simulink model "car_model_FIXED"  (R2022b)
settings: Solver=VariableStepAuto  StartTime=0.0  StopTime=60  RelTol=1e-3
values from neighbouring files (symbols this model uses):
  ABS_MAX_TORQUE = [25 25 25 25]    [workspace.mat]
  ABS_MAX_TRQ_CMD = 50    [workspace.mat]
  ABS_MIN_TORQUE = [0.01 0.01 0.01 0.01]    [workspace.mat]
  acc_IC = 0    [workspace.mat]
  ACCELERATION_MAX = 30    [workspace.mat]
  ActSuspDutyCycle = 1    [workspace.mat]
  Aeq_left = [0.305756190204 0.308857786592 0.311945941182 0.315020811431 0.318082554689 0.321131328186 0.324167289011 0.327190594103 0.330201400225 0.333199863958 0.336186141681 0.339160389558 ... (261 elements, 1x261)]    [workspace.mat]
  Aeq_right = [-0.961664782545 -0.959835898365 -0.957982924115 -0.956106413788 -0.954206913862 -0.952284963337 -0.950341093764 -0.948375829284 -0.946389686656 -0.944383175301 -0.942356797333 -0.940311047601 ... (261 elements, 1x261)]    [workspace.mat]
  alpha_error = 0.1    [workspace.mat]
  ang_acc_hystersesis = 0.1    [workspace.mat]
  ang_IC = 0    [workspace.mat]
  ang_vel_IC = 0    [workspace.mat]
  area_air = 0.15    [workspace.mat]
  axb = -5    [workspace.mat]
  battery_current_IC = 0    [workspace.mat]
  BATTERY_CURRENT_MAX = 140    [workspace.mat]
  BATTERY_CURRENT_MIN = 0    [workspace.mat]
  battery_FT_IC = 300    [workspace.mat]
  battery_T_IC = 300    [workspace.mat]
  BATTERY_TEMPERATURE_MAX = 60    [workspace.mat]
  BATTERY_TEMPERATURE_MIN = 0    [workspace.mat]
  battery_voltage_IC = 332    [workspace.mat]
  BATTERY_VOLTAGE_MAX = 340    [workspace.mat]
  BATTERY_VOLTAGE_MIN = 60    [workspace.mat]
  br = 0.01    [workspace.mat]
  brake_bias = [0.35 0.35 0.15 0.15]    [workspace.mat]
  Brake_Pressure_IC = 1    [workspace.mat]
  ccl_IC = 0    [workspace.mat]
  CENTER_STEER_ANGLE_MAX = 130    [workspace.mat]
  covarience_matrix_IC = [0.001 0 0 0 0 0 0 0 0 0 0 0 ... (784 elements, 28x28)]    [workspace.mat]
  CURRENT_BUFFER = 25    [workspace.mat]
  cy_sweep = [13568.4166816 14020.2069783 14456.754831 14879.7402576 15289.7264712 15687.2766846 16072.954111 16447.3219632 16810.9434544 17164.3817975 17508.2002054 17842.9618912 ... (101 elements, 1x101)]    [workspace.mat]
  dB = 0.001    [workspace.mat]
  dcl_IC = 140    [workspace.mat]
  DCL_MAX = 130    [workspace.mat]
  DCL_MIN = 0    [workspace.mat]
  deadband_angle = 12    [workspace.mat]
  dIndex = 50    [workspace.mat]
  driver_t = 0.015    [workspace.mat]
  dt_OFF = 4.5    [workspace.mat]
  dt_ON = 7.5    [workspace.mat]
  dTx = 0.01    [workspace.mat]
  dx = 0.1    [workspace.mat]
  dZ = 0.295    [workspace.mat]
  efficiency_grid = [0.759500051293 0.787587791453 0.809832189108 0.826747821898 0.837164543102 0.842744381136 0.842258400104 0.838611650621 0.82826195101 0.814029316176 0.795690627225 0.7759791486 ... (2782 elements, 26x107)]    [workspace.mat]
  F0z = [0 0]    [workspace.mat]
  forward_look_straight = 5    [workspace.mat]
  forward_look_turn = 15    [workspace.mat]
  Fz_IC = 539.55    [workspace.mat]
  Fz_sweep = [200 210 220 230 240 250 260 270 280 290 300 310 ... (101 elements, 1x101)]    [workspace.mat]
  g = 9.81    [workspace.mat]
  GAIN_ABS = 100    [workspace.mat]
  gearbox_efficiency = [0.8 0.8 0.8 0.8]    [workspace.mat]
  gps_counter_IC = 0    [workspace.mat]
  gps_hz = 0.01    [workspace.mat]
  gr = [8.74786324786 8.74786324786 8.74786324786 8.74786324786]    [workspace.mat]
  I = 0    [workspace.mat]
  I_Driver = 1    [workspace.mat]
  indicies = [3 3.5 4 0.5 1 1.5 2 2.5 3 3.5 4 0.5 ... (27 elements, 1x27)]    [workspace.mat]
  IYY = 0.3    [workspace.mat]
  kx_sweep = [8779.958 9178.302 9576.646 9974.99 10373.334 10771.678 11170.022 11568.366 11966.71 12365.054 12763.398 13161.742 ... (101 elements, 1x101)]    [workspace.mat]
  l = [0.772 0.772]    [workspace.mat]
  lambda_star = 0.15    [workspace.mat]
  low_V_SA = 0.001    [workspace.mat]
  lr = 35    [workspace.mat]
  m_all = 220    [workspace.mat]
  m_body = 180    [workspace.mat]
  m_unsprung = [6 6 14 14]    [workspace.mat]
  MAG_MAX = 200    [workspace.mat]
  Max_Brake_Pressure = 100000000    [workspace.mat]
  Max_Driver_Input = 1    [workspace.mat]
  MAX_DTHETA_DRIVER = 360    [workspace.mat]
  MAX_I_Driver = 1    [workspace.mat]
  MAX_STEERING_ADJUST = 15    [workspace.mat]
  max_yaw = [0.705271610162 0.928228152446 1.12280857731 1.14131008363 1.08727026041 1.01377803859 0.938114723816 0.8718206875 0.815009168116 0.767481919497 0.727119764215 0.694403589394 ... (15 elements, 1x15)]    [workspace.mat]
  Min_Brake_Pressure = 1    [workspace.mat]
  Min_Driver_Input = 0    [workspace.mat]
  min_velocity_regen = 1.4    [workspace.mat]
  motor_current_IC = 0    [workspace.mat]
  MOTOR_CURRENT_MAX = 70    [workspace.mat]
  MOTOR_CURRENT_MIN = 0    [workspace.mat]
  MOTOR_ENABLE = [0 0 1 1]    [workspace.mat]
  motor_FT_IC = 300    [workspace.mat]
  motor_T_IC = 300    [workspace.mat]
  MOTOR_TEMPERATURE_MAX = 100    [workspace.mat]
  MOTOR_TEMPERATURE_MIN = 0    [workspace.mat]
  motor_voltage_IC = 332    [workspace.mat]
  MOTOR_VOLTAGE_MAX = 340    [workspace.mat]
  MOTOR_VOLTAGE_MIN = 90    [workspace.mat]
  motorControllerCurve = [25  260; 50  130; 75  0]    [workspace.mat]
  motorTempCurve = [140 138.6 134.4 127.4 117.6 105 89.6 71.4 50.4 26.6 0]    [workspace.mat]
  motorTempX = [75 77 79 81 83 85 87 89 91 93 95]    [workspace.mat]
  mu_star = 0.5    [workspace.mat]
  mx_sweep = [3.38348 3.3655067 3.3477908 3.3303323 3.3131312 3.2961875 3.2795012 3.2630723 3.2469008 3.2309867 3.21533 3.1999307 ... (101 elements, 1x101)]    [workspace.mat]
  my_sweep = [3.036232 3.015241699 2.994987032 2.975452753 2.956623616 2.938484375 2.921019784 2.904214597 2.888053568 2.872521451 2.857603 2.843282969 ... (101 elements, 1x101)]    [workspace.mat]
  noise_state = [1e-06 1e-06 1e-06 1e-06 0.005 0.005 0.005 1e-06 1e-06 1e-06 1e-06 1e-06 ... (28 elements, 28x1)]    [workspace.mat]
  omega_IC = 0    [workspace.mat]
  OMEGA_MAX = 150    [workspace.mat]
  OMEGA_MIN = 0    [workspace.mat]
  ORIENTATION_MAX = 360    [workspace.mat]
  P = 2    [workspace.mat]
  P_Driver = 0.7    [workspace.mat]
  P_High_Speed = 0.1    [workspace.mat]
  P_Steering_Adjust = 2    [workspace.mat]
  P_Straight_Adjust = 5    [workspace.mat]
  pos_IC = 0    [workspace.mat]
  POS_MAX = 300    [workspace.mat]
  q_thresh = 0.3    [workspace.mat]
  RE = 0.223    [workspace.mat]
  rho = 1.225    [workspace.mat]
  s = [0.649 0.621]    [workspace.mat]
  selected_maxvm = [49.86390724 16.21289794 8.219813569 8.05215527 7.103352929 8.35634983 13.87515039 8.72402841 22.75224945 36.67909339 19.32001297 25.09036962 ... (63 elements, 21x3)]    [workspace.mat]
  selected_sweep = [3 3 3 3 3 3 3 3 3 3 3 3 ... (1288 elements, 644x2)]    [workspace.mat]
  selected_track = [inf inf inf inf inf inf inf inf inf inf inf inf ... (37971 elements, 4219x9)]    [workspace.mat]
  shock_length_IC = 0.1    [workspace.mat]
  SHOCK_LENGTH_MAX = 0.25    [workspace.mat]
  SHOCK_LENGTH_MIN = 0    [workspace.mat]
  state_IC = [1 0 0 0 0 0 0 0 0 0 0 0 ... (28 elements, 28x1)]    [workspace.mat]
  steering_sweep = [0 5 10 15 20 25 30 35 40 45 50 55 ... (27 elements, 1x27)]    [workspace.mat]
  steering_Up_Grid = [0.551231966244 8.36038106007 16.1333806643 23.9559539118 31.8240691982 39.7561724339 47.7157531433 55.7845698794 64.1341708168 73.0798046026 82.7903081349 93.1297322155 ... (615 elements, 41x15)]    [workspace.mat]
  ... (+25 more)
undefined symbols (not defined in the file or in its folder): ax, ay, az, covA, covG, covM, covP, covV, DiscIntNeverNeededParam, fusion_t, fusion_t_sim, gps_ratio, IMU_accel, IMU_gyro, imu_hz, IMU_mag, location_lla_IC, p, phi, psi, q, r, sus, theta, trn, veh, VEH, whl, X, Xdot, Y, Ydot, Z, Zdot
libraries: fl_lib x82, nesl_utility x32, vehdynlibtire x10, vehdynlibsuspension x8, simulink x5, autolibutils x5, sharedtransform x5, sdl_lib x4, EngineCoolingComponents_lib x4, slpidlib x3, SimscapeFluids_lib x3, shared6dof x2
(part 1 of 14)
settings Model: SimulationMode=accelerator  TunableVars=covA,covM,covP,covV,covG,phi,ref_location,ref_mag_field,location_lla_IC,gps_ratio,noise_state,fusion_t,ABS_MAX_TORQUE,MOTOR_ENABLE,BATTERY_CURRENT_MAX,deadband_angle,alpha_error,I,P,Torque_Up_Rate_Limit,Torque_Down_Rate_Limit,CURRENT_BUFFER,TVS_Intensity  TunableVarsStorageClass=Auto,Auto,Auto,Auto,Auto,Auto,Auto,Auto,Auto,Auto,Auto,Auto,Auto,Auto,Auto,Auto,Auto,Auto,Auto,Auto,Auto,Auto,Auto  TunableVarsTypeQualifier=,,,,,,,,,,,,,,,,,,,,,,  Creator=Inver  LastModifiedBy=Inver
settings DataIOCC: SaveFormat=StructureWithTime  SaveOutput=off  DSMLogging=off
settings OptimizationCC: DefaultParameterBehavior=Inlined  UseDivisionForNetSlopeComputation=on  GainParamInheritBuiltInType=on  UseFloatMulNetSlope=on  InlineInvariantSignals=on  PassReuseOutputArgsAs=Individual arguments  ZeroExternalMemoryAtStartup=off  ZeroInternalMemoryAtStartup=off  NoFixptDivByZeroProtection=on  EfficientFloat2IntCast=on  LifeSpan=1  OptimizeBlockOrder=speed  DifferentSizesBufferReuse=on  EfficientTunableParamExpr=on
settings DebuggingCC: SignalRangeChecking=warning  ReadBeforeWriteMsg=DisableAll  WriteAfterWriteMsg=DisableAll  WriteAfterReadMsg=DisableAll  MultiTaskDSMMsg=none  ParameterTunabilityLossMsg=error  UnderSpecifiedDataTypeMsg=warning  UnderSpecifiedDimensionMsg=warning
settings HardwareCC: ProdBitPerPointer=32  ProdBitPerSizeT=32  ProdBitPerPtrDiffT=32  ProdLargestAtomicInteger=Long  ProdLargestAtomicFloat=Double  ProdWordSize=32  ProdLongLongMode=on  ProdHWDeviceType=ARM Compatible->ARM Cortex-M
settings ModelReferenceCC: EnableRefExpFcnMdlSchedulingChecks=on
settings SFSimCC: SimCustomHeaderCode="#include \"simplex.h\""  SimUserSources=C_Code/simplex.c  SFSimEcho=off  MATLABDynamicMemAlloc=off
settings RTWCC: Description=Embedded Coder  SystemTargetFile=ert.tlc  TemplateMakefile=ert_default_tmf  Toolchain=GNU Tools for ARM Embedded Processors
settings CodeAppCC: ForceParamTrailComments=on  IgnoreCustomStorageClasses=off  OperatorAnnotations=on  SimulinkDataObjDesc=on  SFDataObjDesc=on  CustomSymbolStrGlobalVar=rt$N$M  CustomSymbolStrType=$N$M  CustomSymbolStrFcn=$N$M$F  CustomSymbolStrMacro=$N$M  InsertBlockDesc=on
settings ERTTargetCC: TargetLangStandard=C99 (ISO)  GenerateSampleERTMain=on  IncludeMdlTerminateFcn=off  CombineSignalStateStructs=on  CodeInterfacePackaging=Reusable function  SupportComplex=off  SupportNonInlinedSFcns=on  InlinedParameterPlacement=NonHierarchical  RootIOFormat=Structure reference  ERTCustomFileTemplate=example_file_process.tlc  ERTFilePackagingFormat=CompactWithDataFile

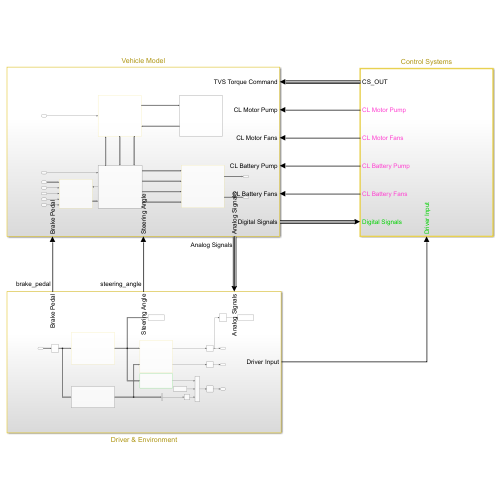
[thumbnail: Simulink's stored preview of the top-level diagram]
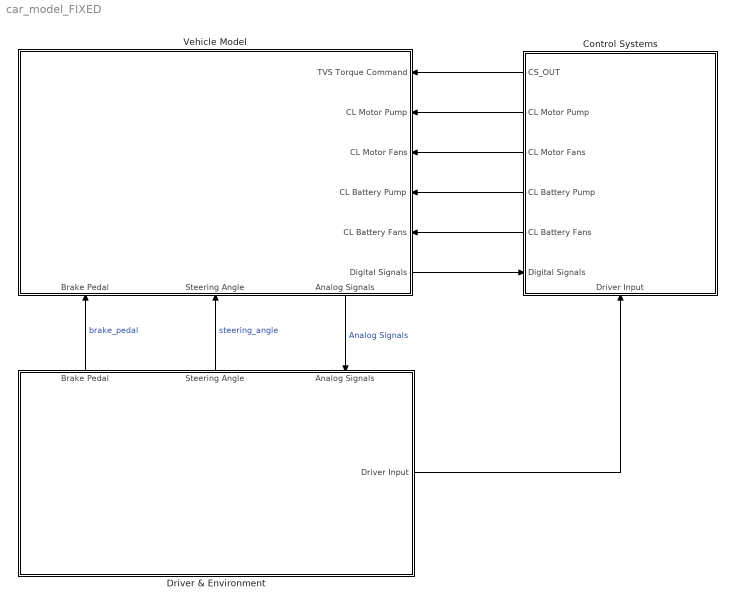
== system car_model_FIXED ==
  Control Systems : Subsystem  TreatAsAtomicUnit=on  RTWFcnName=TVS_SYSTEM  RTWFileName=TVS_SYSTEM
      settings: PortSchema="{\"entries\":[{\"content\":{\"sides\":[{\"content\":{\"connectorIds\":[\"Out1\",\"Out2\",\"Out3\",\"Out4\",\"Out5\",\"In1\"]},\"type\":\"ConnectorPlacement.EquallySpacedRectSide\",\"uuid\":\"b5513b79-39cc-4156-8758-e9dd7d224c4f\"},{\"content\":{\"connectorIds\":[],\"side\":\"RIGHT\"},\"type\":\"ConnectorPlacement.EquallySpacedRectSide\",\"uuid\":\"18919d17-351d-4641-ab2c-66cbba916b4f\"},{\"content\":{\"connectorIds\":[],\"side\":\"TOP\"},\"type\":\"ConnectorPlacement.EquallySpacedRectSide\",\"uuid\":\"63240dfa-789e-427a-a529-4bce5e7f3f10\"},{\"content\":{\"connectorIds\":[\"In2\"],\"side\":\"BOTTOM\"},\"type\":\"ConnectorPlacement.EquallySpacedRectSide\",\"uuid\":\"43cc723f-5f4e-4e66-a14e-4ae2f3e16f9e\"}]},\"type\":\"ConnectorPlacement.EquallySpacedConnector\",\"uuid\":\"47be9ba7-cea3-4b3b-9ee6-e23e075e553b\"}],\"packageUris\":[\"http://schema.mathworks.com/mf0/Connector/R2020b\"],\"version\":\"1.0\"}"
  Driver & Environment : Subsystem
      settings: PortSchema="{\"entries\":[{\"content\":{\"sides\":[{\"content\":{\"connectorIds\":[]},\"type\":\"ConnectorPlacement.EquallySpacedRectSide\",\"uuid\":\"bd499254-800d-4f65-9d66-206e4f6126a9\"},{\"content\":{\"connectorIds\":[\"Out1\"],\"side\":\"RIGHT\"},\"type\":\"ConnectorPlacement.EquallySpacedRectSide\",\"uuid\":\"787bb70a-048d-46a8-9404-9c629bdce5fb\"},{\"content\":{\"connectorIds\":[\"Out2\",\"Out3\",\"In1\"],\"side\":\"TOP\"},\"type\":\"ConnectorPlacement.EquallySpacedRectSide\",\"uuid\":\"94a1f635-0878-46b0-949b-f2a3fa746134\"}]},\"type\":\"ConnectorPlacement.EquallySpacedConnector\",\"uuid\":\"f81a85a8-63b1-46ab-bae2-7f37115d6b57\"}],\"packageUris\":[\"http://schema.mathworks.com/mf0/Connector/R2020b\"],\"version\":\"1.0\"}"
  Vehicle Model : Subsystem
      settings: PortSchema="{\"entries\":[{\"content\":{\"sides\":[{\"content\":{\"connectorIds\":[]},\"type\":\"ConnectorPlacement.EquallySpacedRectSide\",\"uuid\":\"7263df3d-11c2-488e-998f-6bd776306b9c\"},{\"content\":{\"connectorIds\":[\"In3\",\"In4\",\"In5\",\"In6\",\"In7\",\"Out1\"],\"side\":\"RIGHT\"},\"type\":\"ConnectorPlacement.EquallySpacedRectSide\",\"uuid\":\"b0de89c2-35d2-4c59-81fc-f1f509ccf522\"},{\"content\":{\"connectorIds\":[],\"side\":\"TOP\"},\"type\":\"ConnectorPlacement.EquallySpacedRectSide\",\"uuid\":\"474ba072-8402-41d1-8015-97ca573757b9\"},{\"content\":{\"connectorIds\":[\"In1\",\"In2\",\"Out2\"],\"side\":\"BOTTOM\"},\"type\":\"ConnectorPlacement.EquallySpacedRectSide\",\"uuid\":\"2efad9e8-b0d8-4de5-bddc-0b63eaa22f81\"}]},\"type\":\"ConnectorPlacement.EquallySpacedConnector\",\"uuid\":\"426f55ca-7f3f-41f0-94e6-91e6d6304a5e\"}],\"packageUris\":[\"http://schema.mathworks.com/mf0/Connector/R2020b\"],\"version\":\"1.0\"}"
  wires:
  Control Systems/1(CS_OUT) -> Vehicle Model/3(TVS Torque Command)
  Driver & Environment/2(Brake Pedal) -> Vehicle Model/1(Brake Pedal)  "brake_pedal"
  Driver & Environment/3(Steering Angle) -> Vehicle Model/2(Steering Angle)  "steering_angle"
  Vehicle Model/2(Analog Signals) -> Driver & Environment/1(Analog Signals)  "Analog Signals"
  Vehicle Model/1(Digital Signals) -> Control Systems/1(Digital Signals)
  Driver & Environment/1(Driver Input) -> Control Systems/2(Driver Input)
  Control Systems/2(CL Motor Pump) -> Vehicle Model/4(CL Motor Pump)
  Control Systems/4(CL Battery Pump) -> Vehicle Model/6(CL Battery Pump)
  Control Systems/3(CL Motor Fans) -> Vehicle Model/5(CL Motor Fans)
  Control Systems/5(CL Battery Fans) -> Vehicle Model/7(CL Battery Fans)

== system car_model_FIXED/Control Systems ==
  Digital Signals : Inport
  Driver Input : Inport  Port=2
  Bus Creator : BusCreator  Inputs=9
  Bus Creator_boundary_DTC{,1..8} (9 alike) : DataTypeConversion
  Bus Selector : BusSelector  OutputSignals=Corner Dynamics Sensors.theta,Corner Dynamics Sensors.omega,Power Sensors.pwr_lmt,Power Sensors.motor_V,Power Sensors.motor_I,Power Sensors.battery_V,Power Sensors.battery_I,Cooling Sensors.motor_T,Cooling Sensors.mc_T
  Bus Selector1 : BusSelector  OutputSignals=Navigation Sensors.mag,Navigation Sensors.gyro,Navigation Sensors.acc,Navigation Sensors.pos,Navigation Sensors.vel
  Bus Selector2 : BusSelector  OutputSignals=angvel_VNED,vel_VNED
  Bus Selector3 : BusSelector  OutputSignals=Cooling Sensors.motor_T,Cooling Sensors.motor_FT,Cooling Sensors.batt_T,Cooling Sensors.batt_FT
  Bus Selector4 : BusSelector  OutputSignals=Corner Dynamics Sensors.shock_L,Corner Dynamics Sensors.FZ
  CLC : Subsystem
  NFE : Subsystem
  Sensor Fusion : Subsystem  TreatAsAtomicUnit=on  SystemSampleTime=fusion_t_sim
  Sensor Fusion_boundary_DTC{,1..4} (5 alike) : DataTypeConversion
  TV Output Bus : BusCreator  Inputs=18
  TVS : Subsystem  TreatAsAtomicUnit=on  SystemSampleTime=tvs_t_sim
  To Workspace : ToWorkspace  VariableName=TV_Output  SaveFormat=Timeseries  SampleTime=-1
  To Workspace2 : ToWorkspace  VariableName=Sensor_Fused  SaveFormat=Timeseries  SampleTime=-1
  CS_OUT : Outport
  CL Motor Pump : Outport  Port=2
  CL Motor Fans : Outport  Port=3
  CL Battery Pump : Outport  Port=4
  CL Battery Fans : Outport  Port=5
  wires:
  Digital Signals/1 -> Bus Selector3/1, Bus Selector1/1, Bus Selector4/1, Bus Selector/1
  Bus Selector4/1 -> NFE/1(shock_L)  "<shock_L>"
  Bus Selector3/1 -> CLC/1(motor_temperature)  "<motor_T>"
  Bus Selector3/2 -> CLC/2(motor_fluid_temperature)  "<motor_FT>"
  Bus Selector3/3 -> CLC/3(battery_temperature)  "<batt_T>"
  Bus Selector3/4 -> CLC/4(battery_fluid_temperature)  "<batt_FT>"
  CLC/1(CL Motor Pump) -> CL Motor Pump/1
  CLC/2(CL Battery Pump) -> CL Battery Pump/1
  CLC/3(CL Motor Fans) -> CL Motor Fans/1
  CLC/4(CL Battery Fans) -> CL Battery Fans/1
  Bus Selector4/2 -> NFE/2(<Fz>)  "<FZ>"
  Bus Creator/1 -> To Workspace2/1, Bus Selector2/1
  TV Output Bus/1 -> To Workspace/1, CS_OUT/1
  Driver Input/1 -> TVS/1(driver_input)
  NFE/1(Fz) -> TVS/11(Fz)
  Bus Selector2/1 -> TVS/12(angvel_VNED)  "<angvel_VNED>"
  TVS/1(ref_yaw) -> TV Output Bus/1  "ref_yaw"
  TVS/2(beq) -> TV Output Bus/2  "beq"
  TVS/3(obj_gain) -> TV Output Bus/3  "obj_gain"
  TVS/4(lb) -> TV Output Bus/4  "lb"
  TVS/5(ub) -> TV Output Bus/5  "ub"
  TVS/6(windup) -> TV Output Bus/6  "windup"
  TVS/7(Aeq) -> TV Output Bus/7  "Aeq"
  TVS/8(b) -> TV Output Bus/8  "b"
  TVS/10(Tx) -> TV Output Bus/10  "Tx"
  TVS/11(bigM_flag) -> TV Output Bus/11  "bigM_flag"
  TVS/12(omega_m_TV) -> TV Output Bus/12  "omega_m"
  TVS/13(max_ang_acc) -> TV Output Bus/13  "max_ang_acc"
  TVS/14(min_ang_acc) -> TV Output Bus/14  "min_ang_acc"
  TVS/15(motor_I) -> TV Output Bus/15  "motor_I"
  TVS/16(motor_V) -> TV Output Bus/16  "motor_V"
  TVS/17(I_limits) -> TV Output Bus/17  "current_limits"
  TVS/18(batt_V) -> TV Output Bus/18  "battery_V"
  Bus Selector2/2 -> TVS/13(vel_VNED)  "<vel_VNED>"
  Bus Selector/1 -> TVS/2(steering_angle)  "<theta>"
  Bus Selector/2 -> TVS/3(omega)  "<omega>"
  Bus Selector/3 -> TVS/4(current_limits)  "<pwr_lmt>"
  Bus Selector/4 -> TVS/5(motor_voltage)  "<motor_V>"
  Bus Selector/5 -> TVS/6(motor_current)  "<motor_I>"
  Bus Selector/6 -> TVS/7(battery_voltage)  "<battery_V>"
  Bus Selector/7 -> TVS/8(battery_current)  "<battery_I>"
  Bus Selector/8 -> TVS/9(motor_temp)  "<motor_T>"
  Bus Selector/9 -> TVS/10(mc_temp)  "<mc_T>"
  TVS/9(max_b) -> TV Output Bus/9  "max_b"
  Bus Selector1/1 -> Sensor Fusion_boundary_DTC/1  "<mag>"
  Sensor Fusion_boundary_DTC/1 -> Sensor Fusion/1(mag)
  Bus Selector1/2 -> Sensor Fusion_boundary_DTC1/1  "<gyro>"
  Sensor Fusion_boundary_DTC1/1 -> Sensor Fusion/2(gyro)
  Bus Selector1/3 -> Sensor Fusion_boundary_DTC2/1  "<acc>"
  Sensor Fusion_boundary_DTC2/1 -> Sensor Fusion/3(accel)
  Bus Selector1/4 -> Sensor Fusion_boundary_DTC3/1  "<pos>"
  Sensor Fusion_boundary_DTC3/1 -> Sensor Fusion/4(pos)
  Bus Selector1/5 -> Sensor Fusion_boundary_DTC4/1  "<vel>"
  Sensor Fusion_boundary_DTC4/1 -> Sensor Fusion/5(vel)
  Sensor Fusion/1(angvel_VNED) -> Bus Creator_boundary_DTC/1
  Bus Creator_boundary_DTC/1 -> Bus Creator/1  "angvel_VNED"
  Sensor Fusion/2(ang_NED) -> Bus Creator_boundary_DTC1/1
  Bus Creator_boundary_DTC1/1 -> Bus Creator/2  "ang_NED"
  Sensor Fusion/3(pos_VNED) -> Bus Creator_boundary_DTC2/1
  Bus Creator_boundary_DTC2/1 -> Bus Creator/3  "pos_VNED"
  Sensor Fusion/4(vel_VNED) -> Bus Creator_boundary_DTC3/1
  Bus Creator_boundary_DTC3/1 -> Bus Creator/4  "vel_VNED"
  Sensor Fusion/5(acc_VNED) -> Bus Creator_boundary_DTC4/1
  Bus Creator_boundary_DTC4/1 -> Bus Creator/5  "acc_VNED"
  Sensor Fusion/6(mag_VNED) -> Bus Creator_boundary_DTC5/1
  Bus Creator_boundary_DTC5/1 -> Bus Creator/6  "mag_VNED"
  Sensor Fusion/7(acc_bias_VNED) -> Bus Creator_boundary_DTC6/1
  Bus Creator_boundary_DTC6/1 -> Bus Creator/7  "acc_bias_VNED"
  Sensor Fusion/8(gyro_bias_VNED) -> Bus Creator_boundary_DTC7/1
  Bus Creator_boundary_DTC7/1 -> Bus Creator/8  "gyro_bias_VNED"
  Sensor Fusion/9(mag_bias_VNED) -> Bus Creator_boundary_DTC8/1
  Bus Creator_boundary_DTC8/1 -> Bus Creator/9  "mag_bias_VNED"

== system car_model_FIXED/Driver & Environment ==
  Analog Signals : Inport
  Bus Selector : BusSelector  OutputSignals=Steering Angle
  Constant : Constant  Value=YAW_ENABLE
  Lateral Control : Subsystem
  Longitudinal Control : Subsystem
  Rate Limiter : RateLimiter  RisingSlewLimit=MAX_DTHETA_DRIVER  FallingSlewLimit=-MAX_DTHETA_DRIVER  SampleTimeMode=inherited
  Rate Transition : RateTransition  OutPortSampleTime=driver_t
  Rate Transition11 : RateTransition  Deterministic=off  OutPortSampleTime=fusion_t
  Reference Generator : Subsystem
  Sweep Generator : Subsystem
  Switch : Switch  Criteria=u2 > Threshold  SaturateOnIntegerOverflow=off  InputSameDT=off
  To Workspace : ToWorkspace  VariableName=Reference_Generator  SaveFormat=Timeseries  SampleTime=-1
  To Workspace1 : ToWorkspace  VariableName=Throttle  SaveFormat=Timeseries  SampleTime=-1
  Unit Delay : UnitDelay  InitialCondition=Brake_Pressure_IC  SampleTime=driver_t  HasFrameUpgradeWarning=on
  Unit Delay1 : UnitDelay  SampleTime=driver_t  HasFrameUpgradeWarning=on
  Unit Delay2 : UnitDelay  SampleTime=driver_t  HasFrameUpgradeWarning=on
  Driver Input : Outport
  Brake Pedal : Outport  Port=2
  Steering Angle : Outport  Port=3
  wires:
  Longitudinal Control/2(brake_pedal) -> Unit Delay/1  "brake_pressure_pa"
  Lateral Control/1(steering_angle) -> Switch/1  "center_column_steering_angle_deg"
  Longitudinal Control/1(driver_input) -> Unit Delay2/1  "driver_input"
  Switch/1 -> Unit Delay1/1
  Analog Signals/1 -> Rate Transition/1
  Constant/1 -> Switch/2
  Rate Limiter/1 -> Switch/3
  Rate Transition/1 -> Sweep Generator/1(Analog Signals), Reference Generator/1(Analog Signals)
  Unit Delay1/1 -> Steering Angle/1
  Unit Delay2/1 -> Rate Transition11/1, Driver Input/1
  Unit Delay/1 -> Brake Pedal/1
  Reference Generator/1(Controller Information) -> Longitudinal Control/1(Controller Information), To Workspace/1, Lateral Control/1(Controller Information)
  Sweep Generator/1(Controller Information) -> Longitudinal Control/2(Sweep Information), Bus Selector/1
  Bus Selector/1 -> Rate Limiter/1  "<Steering Angle>"
  Rate Transition11/1 -> To Workspace1/1  "throttle"

== system car_model_FIXED/Vehicle Model ==
  Brake Pedal : Inport
  Steering Angle : Inport  Port=2
  TVS Torque Command : Inport  Port=3
  CL Motor Pump : Inport  Port=4
  CL Motor Fans : Inport  Port=5
  CL Battery Pump : Inport  Port=6
  CL Battery Fans : Inport  Port=7
  Electronics : Subsystem
  Powertrain : Subsystem
      settings: PortSchema="{\"entries\":[{\"content\":{\"sides\":[{\"content\":{\"connectorIds\":[\"In1\",\"In2\",\"In3\",\"In4\",\"In5\"]},\"type\":\"ConnectorPlacement.EquallySpacedRectSide\",\"uuid\":\"895a90fc-946f-4344-af69-c005acf2f614\"},{\"content\":{\"connectorIds\":[\"In6\",\"Out1\"],\"side\":\"RIGHT\"},\"type\":\"ConnectorPlacement.EquallySpacedRectSide\",\"uuid\":\"931fcb49-b75e-480c-a4d6-2f82b080d057\"},{\"content\":{\"connectorIds\":[],\"side\":\"TOP\"},\"type\":\"ConnectorPlacement.EquallySpacedRectSide\",\"uuid\":\"d1b12b51-387e-4553-b5da-149d57232505\"}]},\"type\":\"ConnectorPlacement.EquallySpacedConnector\",\"uuid\":\"0cb2c3dd-4627-421c-9ed4-7e8c572a9937\"}],\"packageUris\":[\"http://schema.mathworks.com/mf0/Connector/R2020b\"],\"version\":\"1.0\"}"
  Suspension : Subsystem  Variant=on  VariantControlMode=label  LabelModeActiveChoice=1
      settings: PortSchema="{\"entries\":[{\"content\":{\"sides\":[{\"content\":{\"connectorIds\":[\"In1\"]},\"type\":\"ConnectorPlacement.EquallySpacedRectSide\",\"uuid\":\"d90bf910-501d-4dd1-a367-d76bd42ab174\"},{\"content\":{\"connectorIds\":[\"Out1\",\"In3\"],\"side\":\"RIGHT\"},\"type\":\"ConnectorPlacement.EquallySpacedRectSide\",\"uuid\":\"1fe7da07-1086-4d5e-8baf-d5d069455d6e\"},{\"content\":{\"connectorIds\":[],\"side\":\"TOP\"},\"type\":\"ConnectorPlacement.EquallySpacedRectSide\",\"uuid\":\"6ff63b9e-45bb-47e9-90cd-47f8e0815e57\"},{\"content\":{\"connectorIds\":[\"In2\",\"Out2\",\"Out3\"],\"side\":\"BOTTOM\"},\"type\":\"ConnectorPlacement.EquallySpacedRectSide\",\"uuid\":\"116c6de0-7bfa-4dc1-bfd0-57a2fffb3aa0\"}]},\"type\":\"ConnectorPlacement.EquallySpacedConnector\",\"uuid\":\"6475b998-12b0-4b0e-8a20-c379b8e08c7c\"}],\"packageUris\":[\"http://schema.mathworks.com/mf0/Connector/R2020b\"],\"version\":\"1.0\"}"
      mask Display:
      | switch str2num(get_param(gcb,'ActiveVariant'))
      |     case 1
      |         image('suspdw.png');
      |     case 2
      |         image([imread('suspindmap.png');imread('suspsamap.png')]);
      |     case 3
      |          image([imread('suspmacp.png');imread('suspsacoil.png')]);
      |     case 4
      |          image('suspmacp.png');
      |     case 5
      |          image('suspindmap.png');
      |     case 6
      |          image('suspkandc.png');
      | end
  Vehicle : Subsystem
      settings: PortSchema="{\"entries\":[{\"content\":{\"sides\":[{\"content\":{\"connectorIds\":[\"In1\",\"Out1\"]},\"type\":\"ConnectorPlacement.EquallySpacedRectSide\",\"uuid\":\"63fa377f-0583-4c60-bac7-9bd73dadd9a1\"},{\"content\":{\"connectorIds\":[],\"side\":\"RIGHT\"},\"type\":\"ConnectorPlacement.EquallySpacedRectSide\",\"uuid\":\"7f668e34-aa5e-4f2f-9be8-80fbb83ff2c8\"},{\"content\":{\"connectorIds\":[],\"side\":\"TOP\"},\"type\":\"ConnectorPlacement.EquallySpacedRectSide\",\"uuid\":\"511f439c-568f-45f1-9ff4-54e644eb8180\"}]},\"type\":\"ConnectorPlacement.EquallySpacedConnector\",\"uuid\":\"b54bf87e-fa06-468b-8fa9-38148d60ed3d\"}],\"packageUris\":[\"http://schema.mathworks.com/mf0/Connector/R2020b\"],\"version\":\"1.0\"}"
      mask Display: image('6dofcar.png');
  Wheels and Tires : Subsystem
      settings: PortSchema="{\"entries\":[{\"content\":{\"sides\":[{\"content\":{\"connectorIds\":[\"In1\",\"Out6\",\"In2\"]},\"type\":\"ConnectorPlacement.EquallySpacedRectSide\",\"uuid\":\"77263124-783e-4307-b979-a6212540af24\"},{\"content\":{\"connectorIds\":[\"Out1\",\"Out2\",\"Out3\",\"Out4\"],\"side\":\"RIGHT\"},\"type\":\"ConnectorPlacement.EquallySpacedRectSide\",\"uuid\":\"cb03b446-69c2-4dbf-929b-d33818acfe8b\"},{\"content\":{\"connectorIds\":[\"Out5\",\"In3\",\"In4\"],\"side\":\"TOP\"},\"type\":\"ConnectorPlacement.EquallySpacedRectSide\",\"uuid\":\"8e7e4023-62e5-48a8-8666-b4c8bb14cd01\"}]},\"type\":\"ConnectorPlacement.EquallySpacedConnector\",\"uuid\":\"1061f0db-ec8e-49bd-8d66-b4a53eaeacfa\"}],\"packageUris\":[\"http://schema.mathworks.com/mf0/Connector/R2020b\"],\"version\":\"1.0\"}"
      mask Display: image('wheel3dof.png')
  Digital Signals : Outport  PortDimensions={292}
  Analog Signals : Outport  Port=2  PortDimensions={292}
  wires:
  Steering Angle/1 -> Suspension/1(Steering)
  Suspension/1(Suspension) -> Vehicle/1(Suspension)  "Susp"
  Wheels and Tires/5(Wheels2Susp) -> Suspension/2(Wheel)
  Powertrain/1(PwrTrn) -> Wheels and Tires/2(PwrTrn)
  Brake Pedal/1 -> Wheels and Tires/1(Brake Press)
  TVS Torque Command/1 -> Powertrain/1(TVS Torque Command)
  Suspension/2(Suspension1) -> Wheels and Tires/3(Sus)
  Vehicle/1(VehFdbk) -> Suspension/3(Vehicle)  "Vehicle"
  Suspension/3(Veh) -> Wheels and Tires/4(Veh)
  Wheels and Tires/1(Vehicle) -> Electronics/1(Veh)  "veh"
  Wheels and Tires/2(Suspension) -> Electronics/2(Sus)  "sus"
  Wheels and Tires/3(Wheels) -> Electronics/3(Whl)  "whl"
  Electronics/1(Analog Signals) -> Analog Signals/1
  Electronics/2(Digital Signals) -> Digital Signals/1
  Wheels and Tires/4(Power Train) -> Electronics/4(Trn)  "trn"
  CL Motor Pump/1 -> Powertrain/2(CL Motor Pump)
  CL Battery Pump/1 -> Powertrain/4(CL Battery Pump)
  CL Motor Fans/1 -> Powertrain/3(CL Motor Fans)
  CL Battery Fans/1 -> Powertrain/5(CL Battery Fans)
  Wheels and Tires/6(Vg) -> Powertrain/6(Vg)

== system car_model_FIXED/Control Systems/CLC ==
  motor_temperature : Inport
  motor_fluid_temperature : Inport  Port=2
  battery_temperature : Inport  Port=3
  battery_fluid_temperature : Inport  Port=4
  Step : Step  After=0  SampleTime=0
  CL Motor Pump : Outport
  CL Battery Pump : Outport  Port=2
  CL Motor Fans : Outport  Port=3
  CL Battery Fans : Outport  Port=4
  wires:
  Step/1 -> CL Motor Fans/1, CL Battery Fans/1, CL Battery Pump/1, CL Motor Pump/1

== system car_model_FIXED/Control Systems/NFE ==
  shock_L : Inport
  <Fz> : Inport  Port=2
  Saturation17 : Saturate  UpperLimit=1200  LowerLimit=200
  Terminator : Terminator
  Fz : Outport
  wires:
  shock_L/1 -> Terminator/1
  <Fz>/1 -> Saturation17/1
  Saturation17/1 -> Fz/1  "FZ"

== system car_model_FIXED/Control Systems/Sensor Fusion ==
  mag : Inport  OutMin=-MAG_MAX  OutMax=MAG_MAX
  gyro : Inport  Port=2  OutMin=-YAW_MAX  OutMax=YAW_MAX
  accel : Inport  Port=3  OutMin=-ACCELERATION_MAX  OutMax=ACCELERATION_MAX
  pos : Inport  Port=4  OutMin=-POS_MAX  OutMax=POS_MAX
  vel : Inport  Port=5  OutMin=-VELOCITY_MAX  OutMax=VELOCITY_MAX
  NED2VNED : MATLAB Function  TreatAsAtomicUnit=on
  SNED to VNED : MATLAB Function  TreatAsAtomicUnit=on
  Transpose{,1..11} (12 alike) : Math  Operator=transpose
  Unit Delay1 : UnitDelay  InitialCondition=gps_counter_IC  SampleTime=-1  HasFrameUpgradeWarning=on
  Unit Delay2 : UnitDelay  InitialCondition=state_IC  SampleTime=-1  HasFrameUpgradeWarning=on
  Unit Delay3 : UnitDelay  InitialCondition=covarience_matrix_IC  SampleTime=-1  HasFrameUpgradeWarning=on
  fusion : MATLAB Function  TreatAsAtomicUnit=on
  angvel_VNED : Outport  OutMin=-YAW_MAX  OutMax=YAW_MAX
  ang_NED : Outport  Port=2  OutMin=-1  OutMax=1
  pos_VNED : Outport  Port=3  OutMin=-POS_MAX  OutMax=POS_MAX
  vel_VNED : Outport  Port=4  OutMin=-VELOCITY_MAX  OutMax=VELOCITY_MAX
  acc_VNED : Outport  Port=5  OutMin=-ACCELERATION_MAX  OutMax=ACCELERATION_MAX
  mag_VNED : Outport  Port=6  OutMin=-MAG_MAX  OutMax=MAG_MAX
  acc_bias_VNED : Outport  Port=7  OutMin=-ACCELERATION_MAX  OutMax=ACCELERATION_MAX
  gyro_bias_VNED : Outport  Port=8  OutMin=-YAW_MAX  OutMax=YAW_MAX
  mag_bias_VNED : Outport  Port=9  OutMin=-MAG_MAX  OutMax=MAG_MAX
  wires:
  NED2VNED/7(accel_bias) -> Transpose8/1  "acc_bias_VNED"
  NED2VNED/3(pos) -> Transpose9/1  "pos_VNED"
  NED2VNED/4(vel) -> Transpose5/1  "vel_VNED"
  NED2VNED/2(angvel) -> Transpose10/1  "angvel_VNED"
  NED2VNED/1(ang) -> Transpose11/1  "ang_NED"
  fusion/2(rot_map) -> NED2VNED/1(rot_map)
  Transpose/1 -> fusion/4(acceleration)
  Unit Delay3/1 -> fusion/8(cov_in)
  NED2VNED/8(gyro_bias) -> Transpose4/1  "gyro_bias_VNED"
  Transpose1/1 -> fusion/5(angularVelocity)
  fusion/4(cov_out) -> Unit Delay3/1
  fusion/3(state_out) -> Unit Delay2/1, NED2VNED/2(state)
  SNED to VNED/2(gyro_VNED) -> Transpose1/1  "gyro_VNED"
  SNED to VNED/1(accel_VNED) -> Transpose/1  "accel_VNED"
  NED2VNED/5(accel) -> Transpose6/1  "acc_VNED"
  SNED to VNED/3(mag_VNED) -> Transpose2/1  "mag_VNED"
  Unit Delay2/1 -> fusion/7(state_in)
  Transpose2/1 -> fusion/6(magField)
  NED2VNED/9(mag_bias) -> Transpose3/1  "mag_bias_VNED"
  NED2VNED/6(mag) -> Transpose7/1  "mag_VNED"
  accel/1 -> SNED to VNED/1(accel_SNED)
  gyro/1 -> SNED to VNED/2(gyro_SNED)
  mag/1 -> SNED to VNED/3(mag_SNED)
  pos/1 -> fusion/3(position)
  vel/1 -> fusion/2(velocity)
  Transpose3/1 -> mag_bias_VNED/1
  Transpose4/1 -> gyro_bias_VNED/1
  Transpose8/1 -> acc_bias_VNED/1
  Transpose7/1 -> mag_VNED/1
  Transpose6/1 -> acc_VNED/1
  Transpose5/1 -> vel_VNED/1
  Transpose9/1 -> pos_VNED/1
  Transpose10/1 -> angvel_VNED/1
  Transpose11/1 -> ang_NED/1
  fusion/1(count) -> Unit Delay1/1
  Unit Delay1/1 -> fusion/1("count ")

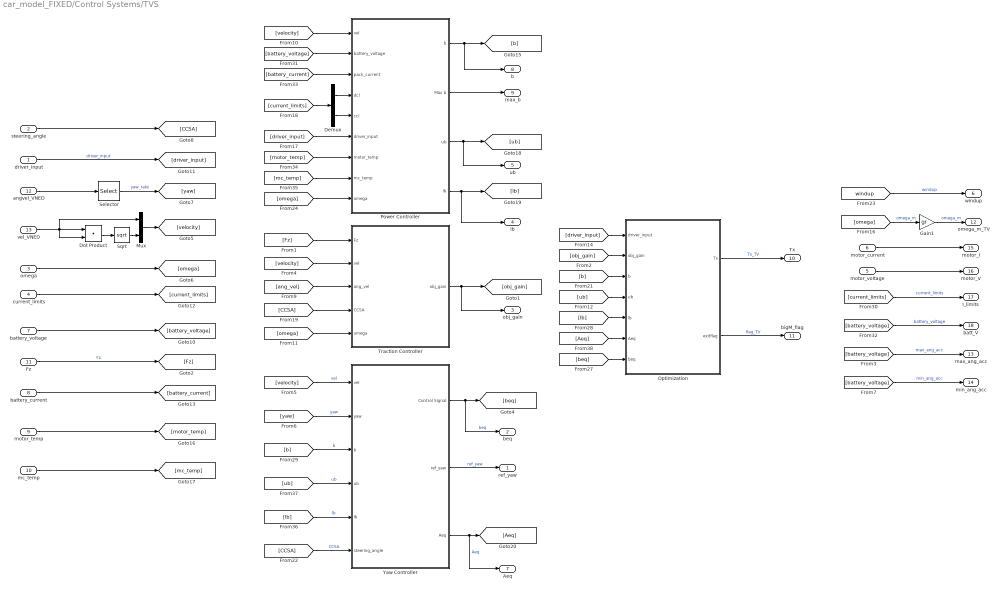
== system car_model_FIXED/Control Systems/TVS ==
  driver_input : Inport  OutMin=-1  OutMax=1  OutDataTypeStr=double  PortDimensions=1  LockScale=on
  steering_angle : Inport  Port=2  OutMin=-130  OutMax=130  OutDataTypeStr=double  PortDimensions=1
  omega : Inport  Port=3  OutMin=0  OutMax=150  OutDataTypeStr=double  LockScale=on
  current_limits : Inport  Port=4  OutMin=-80000  OutMax=80000  OutDataTypeStr=double  LockScale=on
  motor_voltage : Inport  Port=5
  motor_current : Inport  Port=6
  battery_voltage : Inport  Port=7  OutMin=50  OutMax=340  OutDataTypeStr=double
  battery_current : Inport  Port=8
  motor_temp : Inport  Port=9
  mc_temp : Inport  Port=10
  Fz : Inport  Port=11
  angvel_VNED : Inport  Port=12  OutMin=-5  OutMax=5  OutDataTypeStr=double  PortDimensions=[1 3]  LockScale=on
  vel_VNED : Inport  Port=13  OutMin=0  OutMax=30  OutDataTypeStr=double  LockScale=on
  Demux : Demux  Outputs=2
  Dot Product : DotProduct  OutDataTypeStr=Inherit: Inherit via internal rule
  Gain1 : Gain  Gain=gr  ParamDataTypeStr=double  OutDataTypeStr=Inherit: Inherit via back propagation
  Mux : Mux  Inputs=2
  Optimization : Subsystem
  Power Controller : Subsystem
  Selector : Selector  InputPortWidth=3  IndexOptions=Index vector (dialog)  Indices=3  OutputSizes=1
  Sqrt : Sqrt
  Traction Controller : Subsystem
  Yaw Controller : Subsystem
  ref_yaw : Outport
  beq : Outport  Port=2  OutMin=-10  OutMax=10  OutDataTypeStr=double  LockScale=on
  obj_gain : Outport  Port=3
  lb : Outport  Port=4  OutMin=-25  OutMax=25  OutDataTypeStr=double  LockScale=on
  ub : Outport  Port=5  OutMin=-25  OutMax=25  OutDataTypeStr=double  LockScale=on
  windup : Outport  Port=6
  Aeq : Outport  Port=7  OutMin=-1.9  OutMax=1.9  OutDataTypeStr=double  LockScale=on
  b : Outport  Port=8  OutMin=-80000  OutMax=80000  OutDataTypeStr=double  LockScale=on
  max_b : Outport  Port=9  OutMin=-80000  OutMax=80000  OutDataTypeStr=double  LockScale=on
  Tx : Outport  Port=10  OutDataTypeStr=double  PortDimensions=[1 4]
  bigM_flag : Outport  Port=11  PortDimensions=1
  omega_m_TV : Outport  Port=12
  max_ang_acc : Outport  Port=13
  min_ang_acc : Outport  Port=14
  motor_I : Outport  Port=15
  motor_V : Outport  Port=16
  I_limits : Outport  Port=17
  batt_V : Outport  Port=18
  wires:
  motor_current/1 -> motor_I/1
  motor_voltage/1 -> motor_V/1
  omega/1 -> [omega]
  [velocity] -> Traction Controller/2(vel)
  current_limits/1 -> [current_limits]
  Optimization/2(exitflag) -> bigM_flag/1  "flag_TV"
  vel_VNED/1 -> Mux/1, Dot Product/2, Dot Product/1
  [omega] -> Gain1/1  "omega_m"
  [velocity] -> Yaw Controller/1(vel)  "vel"
  [ang_vel] -> Traction Controller/3(ang_vel)
  Power Controller/1(b) -> b/1, [b]
  Traction Controller/1(obj_gain) -> [obj_gain], obj_gain/1
  Power Controller/3(ub) -> [ub], ub/1
  angvel_VNED/1 -> Selector/1
  [omega] -> Traction Controller/5(omega)
  battery_voltage/1 -> [battery_voltage]
  [driver_input] -> Optimization/1(driver_input)
  Yaw Controller/1(Control Signal) -> [beq], beq/1  "beq"
  [yaw] -> Yaw Controller/2(yaw)  "yaw"
  [Fz] -> Traction Controller/1(Fz)
  [windup] -> windup/1  "windup"
  Yaw Controller/3(Aeq) -> [Aeq], Aeq/1  "Aeq"
  driver_input/1 -> [driver_input]  "driver_input"
  [beq] -> Optimization/7(beq)
  Power Controller/4(lb) -> [lb], lb/1
  Fz/1 -> [Fz]  "Fz"
  [obj_gain] -> Optimization/2(obj_gain)
  Yaw Controller/2(ref_yaw) -> ref_yaw/1  "ref_yaw"
  Optimization/1(Tx) -> Tx/1  "Tx_TV"
  [current_limits] -> I_limits/1  "current_limits"
  [battery_voltage] -> batt_V/1  "battery_voltage"
  battery_current/1 -> [battery_current]
  Selector/1 -> [yaw]  "yaw_rate"
  Dot Product/1 -> Sqrt/1
  Mux/1 -> [velocity]
  Sqrt/1 -> Mux/2
  motor_temp/1 -> [motor_temp]
  mc_temp/1 -> [mc_temp]
  Gain1/1 -> omega_m_TV/1  "omega_m"
  steering_angle/1 -> [CCSA]
  [CCSA] -> Traction Controller/4(CCSA)
  [velocity] -> Power Controller/1(vel)
  [battery_voltage] -> Power Controller/2(battery_voltage)
  [battery_current] -> Power Controller/3(pack_current)
  [driver_input] -> Power Controller/6(driver_input)
  [motor_temp] -> Power Controller/7(motor_temp)
  [mc_temp] -> Power Controller/8(mc_temp)
  [current_limits] -> Demux/1
  Demux/2 -> Power Controller/5(ccl)
  Demux/1 -> Power Controller/4(dcl)
  [CCSA] -> Yaw Controller/6(steering_angle)  "CCSA"
  [ub] -> Optimization/4(ub)
  [lb] -> Optimization/5(lb)
  [b] -> Optimization/3(b)
  [ub] -> Yaw Controller/4(ub)  "ub"
  [lb] -> Yaw Controller/5(lb)  "lb"
  [b] -> Yaw Controller/3(b)  "b"
  [Aeq] -> Optimization/6(Aeq)
  [omega] -> Power Controller/9(omega)
  [battery_voltage] -> max_ang_acc/1  "max_ang_acc"
  [battery_voltage] -> min_ang_acc/1  "min_ang_acc"
  Power Controller/2(Max b) -> max_b/1

== system car_model_FIXED/Driver & Environment/Lateral Control ==
  Controller Information : Inport
  1-D Lookup Table : Lookup_n-D  NumberOfTableDimensions=1  BreakpointsForDimension1=velocity_sweep  Table=max_yaw  ExtrapMethod=Clip  InternalRulePriority=Speed  RndMeth=Simplest
  2-D Lookup Table1 : Lookup_n-D  BreakpointsForDimension1=yaw_rate_sweep  BreakpointsForDimension2=velocity_sweep  Table=steering_Up_Grid  ExtrapMethod=Clip  InternalRulePriority=Speed  RndMeth=Simplest
      settings: InputPortMap=u0,u1
  2-D Lookup Table2 : Lookup_n-D  BreakpointsForDimension1=yaw_rate_sweep  BreakpointsForDimension2=velocity_sweep  Table=steering_Up_Grid  ExtrapMethod=Clip  InternalRulePriority=Speed  RndMeth=Simplest
      settings: InputPortMap=u0,u1
  Abs : Abs  SaturateOnIntegerOverflow=off
  Bus Selector : BusSelector  OutputSignals=p_error,Vnow,yaw_ref,v_cog
  Constant : Constant  Value=17.5
  Constant1 : Constant  Value=0
  GreaterThan : RelationalOperator  Operator=>  OutDataTypeStr=boolean  RndMeth=Simplest  InputSameDT=off
  GreaterThan1 : RelationalOperator  Operator=~=  OutDataTypeStr=boolean  RndMeth=Simplest  InputSameDT=off
  Min : MinMax  Inputs=2
  NAND : Logic  Operator=NAND  IconShape=distinctive  AllPortsSameDT=off  OutDataTypeStr=boolean
  NOT : Logic  Operator=NOT  IconShape=distinctive  AllPortsSameDT=off  OutDataTypeStr=boolean
  PID Controller : slpidlib/PID Controller  Controller=PID  Form=Parallel  TimeDomain=Discrete-time  UseExternalTs=off  SampleTime=-1  IntegratorMethod=Forward Euler  FilterMethod=Forward Euler  ControllerParametersSource=internal  P=P_Straight_Adjust  I=0  UseKiTs=on  D=0  N=0  UseFilter=on  TunerSelectOption=Transfer Function Based (PID Tuner App)  InitialConditionSource=internal  InitialConditionForIntegrator=0  InitialConditionForFilter=0  DifferentiatorICPrevScaledInput=0  ExternalReset=none  TrackingMode=off  Kt=1  LimitOutput=on  SatLimitsSource=internal  UpperSaturationLimit=MAX_STEERING_ADJUST  LowerSaturationLimit=-MAX_STEERING_ADJUST  LinearizeAsGain=on  AntiWindupMode=none  Kb=1  LimitIntegrator=off  UpperIntegratorSaturationLimit=inf  LowerIntegratorSaturationLimit=-inf  POutMin=[]  POutMax=[]  IOutMin=[]  IOutMax=[]  DOutMin=[]  DOutMax=[]  NOutMin=[]  NOutMax=[]  SumOutMin=[]  SumOutMax=[]  SaturationOutMin=[]  SaturationOutMax=[]  PParamMin=[]  PParamMax=[]  IParamMin=[]  IParamMax=[]  DParamMin=[]  DParamMax=[]  NParamMin=[]  NParamMax=[]  KbParamMin=[]  KbParamMax=[]  KtParamMin=[]  KtParamMax=[]  KbOutMin=[]  KbOutMax=[]  KtOutMin=[]  KtOutMax=[]  IntegratorOutMin=[]  IntegratorOutMax=[]  FilterOutMin=[]  FilterOutMax=[]  SumI1OutMin=[]  SumI1OutMax=[]  SumI2OutMin=[]  SumI2OutMax=[]  SumI3OutMin=[]  SumI3OutMax=[]  SumI4OutMin=[]  SumI4OutMax=[]  SumDOutMin=[]  SumDOutMax=[]  DifferentiatorOutMin=[]  DifferentiatorOutMax=[]  FilterDiffOutCoefMin=[]  FilterDiffOutCoefMax=[]  ReciprocalOutMin=[]  ReciprocalOutMax=[]  SumDenOutMin=[]  SumDenOutMax=[]  SumNumOutMin=[]  SumNumOutMax=[]  DivideOutMin=[]  DivideOutMax=[]  UdiffTsProdOutMin=[]  UdiffTsProdOutMax=[]  NTsProdOutMin=[]  NTsProdOutMax=[]  UintegralTsProdOutMin=[]  UintegralTsProdOutMax=[]  UngainTsProdOutMin=[]  UngainTsProdOutMax=[]  ClampingZeroOutDataTypeStr=Inherit: Inherit via back propagation  ClampingZeroOutMin=[]  ClampingZeroOutMax=[]  FilterDenConstantOutDataTypeStr=Inherit: Inherit via back propagation  FilterDenConstantOutMin=[]  FilterDenConstantOutMax=[]  PCopyOutDataTypeStr=Inherit: Inherit via back propagation  PCopyOutMin=[]  PCopyOutMax=[]  NCopyOutDataTypeStr=Inherit: Inherit via back propagation  NCopyOutMin=[]  NCopyOutMax=[]  IntegratorContinuousStateAttributes=''  IntegratorStateMustResolveToSignalObject=off  IntegratorRTWStateStorageClass=Auto  FilterContinuousStateAttributes=''  FilterStateMustResolveToSignalObject=off  FilterRTWStateStorageClass=Auto  ParallelPVariant=InternalParameters  IdealPVariant=Disabled  IVariant=InternalParameters  DVariant=InternalParameters  IntegratorVariant=Discrete  SatVariant=Enabled  AWVariant=Passthrough  PCopyVariant=Disabled  TRVariant=Disabled  FdbkBlocksVariant=Forward  IdealPFdbkVariant=Disabled  SatFdbkVariant=Disabled  DerivativeFilterVariant=ForwardEulerFilter  NVariant=InternalParameters  NCopyVariant=Disabled  FilterICVariant=InternalICsFilter  IntegratorICVariant=InternalICs  ExternalResetVariant=Disabled  TRSumVariant=Passthrough  SumFdbkVariant=Disabled  SumVariant=Sum_PID  TsampFilterVariant=InternalTs  TsampNgainVariant=Passthrough  TsampIntegralVariant=Passthrough  ExternalSaturationOutDataTypeStr=Inherit: Same as second input
  PID Controller1 : slpidlib/PID Controller  Controller=PID  Form=Parallel  TimeDomain=Discrete-time  UseExternalTs=off  SampleTime=-1  IntegratorMethod=Forward Euler  FilterMethod=Forward Euler  ControllerParametersSource=internal  P=P_Steering_Adjust  I=0  UseKiTs=on  D=0  N=0  UseFilter=on  TunerSelectOption=Transfer Function Based (PID Tuner App)  InitialConditionSource=internal  InitialConditionForIntegrator=0  InitialConditionForFilter=0  DifferentiatorICPrevScaledInput=0  ExternalReset=none  TrackingMode=off  Kt=1  LimitOutput=on  SatLimitsSource=internal  UpperSaturationLimit=MAX_STEERING_ADJUST  LowerSaturationLimit=-MAX_STEERING_ADJUST  LinearizeAsGain=on  AntiWindupMode=none  Kb=1  LimitIntegrator=off  UpperIntegratorSaturationLimit=inf  LowerIntegratorSaturationLimit=-inf  POutMin=[]  POutMax=[]  IOutMin=[]  IOutMax=[]  DOutMin=[]  DOutMax=[]  NOutMin=[]  NOutMax=[]  SumOutMin=[]  SumOutMax=[]  SaturationOutMin=[]  SaturationOutMax=[]  PParamMin=[]  PParamMax=[]  IParamMin=[]  IParamMax=[]  DParamMin=[]  DParamMax=[]  NParamMin=[]  NParamMax=[]  KbParamMin=[]  KbParamMax=[]  KtParamMin=[]  KtParamMax=[]  KbOutMin=[]  KbOutMax=[]  KtOutMin=[]  KtOutMax=[]  IntegratorOutMin=[]  IntegratorOutMax=[]  FilterOutMin=[]  FilterOutMax=[]  SumI1OutMin=[]  SumI1OutMax=[]  SumI2OutMin=[]  SumI2OutMax=[]  SumI3OutMin=[]  SumI3OutMax=[]  SumI4OutMin=[]  SumI4OutMax=[]  SumDOutMin=[]  SumDOutMax=[]  DifferentiatorOutMin=[]  DifferentiatorOutMax=[]  FilterDiffOutCoefMin=[]  FilterDiffOutCoefMax=[]  ReciprocalOutMin=[]  ReciprocalOutMax=[]  SumDenOutMin=[]  SumDenOutMax=[]  SumNumOutMin=[]  SumNumOutMax=[]  DivideOutMin=[]  DivideOutMax=[]  UdiffTsProdOutMin=[]  UdiffTsProdOutMax=[]  NTsProdOutMin=[]  NTsProdOutMax=[]  UintegralTsProdOutMin=[]  UintegralTsProdOutMax=[]  UngainTsProdOutMin=[]  UngainTsProdOutMax=[]  ClampingZeroOutDataTypeStr=Inherit: Inherit via back propagation  ClampingZeroOutMin=[]  ClampingZeroOutMax=[]  FilterDenConstantOutDataTypeStr=Inherit: Inherit via back propagation  FilterDenConstantOutMin=[]  FilterDenConstantOutMax=[]  PCopyOutDataTypeStr=Inherit: Inherit via back propagation  PCopyOutMin=[]  PCopyOutMax=[]  NCopyOutDataTypeStr=Inherit: Inherit via back propagation  NCopyOutMin=[]  NCopyOutMax=[]  IntegratorContinuousStateAttributes=''  IntegratorStateMustResolveToSignalObject=off  IntegratorRTWStateStorageClass=Auto  FilterContinuousStateAttributes=''  FilterStateMustResolveToSignalObject=off  FilterRTWStateStorageClass=Auto  ParallelPVariant=InternalParameters  IdealPVariant=Disabled  IVariant=InternalParameters  DVariant=InternalParameters  IntegratorVariant=Discrete  SatVariant=Enabled  AWVariant=Passthrough  PCopyVariant=Disabled  TRVariant=Disabled  FdbkBlocksVariant=Forward  IdealPFdbkVariant=Disabled  SatFdbkVariant=Disabled  DerivativeFilterVariant=ForwardEulerFilter  NVariant=InternalParameters  NCopyVariant=Disabled  FilterICVariant=InternalICsFilter  IntegratorICVariant=InternalICs  ExternalResetVariant=Disabled  TRSumVariant=Passthrough  SumFdbkVariant=Disabled  SumVariant=Sum_PID  TsampFilterVariant=InternalTs  TsampNgainVariant=Passthrough  TsampIntegralVariant=Passthrough  ExternalSaturationOutDataTypeStr=Inherit: Same as second input
  PID Controller2 : slpidlib/PID Controller  Controller=PID  Form=Parallel  TimeDomain=Discrete-time  UseExternalTs=off  SampleTime=-1  IntegratorMethod=Forward Euler  FilterMethod=Forward Euler  ControllerParametersSource=internal  P=P_High_Speed  I=0  UseKiTs=on  D=0  N=0  UseFilter=on  TunerSelectOption=Transfer Function Based (PID Tuner App)  InitialConditionSource=internal  InitialConditionForIntegrator=0  InitialConditionForFilter=0  DifferentiatorICPrevScaledInput=0  ExternalReset=none  TrackingMode=off  Kt=1  LimitOutput=on  SatLimitsSource=internal  UpperSaturationLimit=MAX_STEERING_ADJUST  LowerSaturationLimit=-MAX_STEERING_ADJUST  LinearizeAsGain=on  AntiWindupMode=none  Kb=1  LimitIntegrator=off  UpperIntegratorSaturationLimit=inf  LowerIntegratorSaturationLimit=-inf  POutMin=[]  POutMax=[]  IOutMin=[]  IOutMax=[]  DOutMin=[]  DOutMax=[]  NOutMin=[]  NOutMax=[]  SumOutMin=[]  SumOutMax=[]  SaturationOutMin=[]  SaturationOutMax=[]  PParamMin=[]  PParamMax=[]  IParamMin=[]  IParamMax=[]  DParamMin=[]  DParamMax=[]  NParamMin=[]  NParamMax=[]  KbParamMin=[]  KbParamMax=[]  KtParamMin=[]  KtParamMax=[]  KbOutMin=[]  KbOutMax=[]  KtOutMin=[]  KtOutMax=[]  IntegratorOutMin=[]  IntegratorOutMax=[]  FilterOutMin=[]  FilterOutMax=[]  SumI1OutMin=[]  SumI1OutMax=[]  SumI2OutMin=[]  SumI2OutMax=[]  SumI3OutMin=[]  SumI3OutMax=[]  SumI4OutMin=[]  SumI4OutMax=[]  SumDOutMin=[]  SumDOutMax=[]  DifferentiatorOutMin=[]  DifferentiatorOutMax=[]  FilterDiffOutCoefMin=[]  FilterDiffOutCoefMax=[]  ReciprocalOutMin=[]  ReciprocalOutMax=[]  SumDenOutMin=[]  SumDenOutMax=[]  SumNumOutMin=[]  SumNumOutMax=[]  DivideOutMin=[]  DivideOutMax=[]  UdiffTsProdOutMin=[]  UdiffTsProdOutMax=[]  NTsProdOutMin=[]  NTsProdOutMax=[]  UintegralTsProdOutMin=[]  UintegralTsProdOutMax=[]  UngainTsProdOutMin=[]  UngainTsProdOutMax=[]  ClampingZeroOutDataTypeStr=Inherit: Inherit via back propagation  ClampingZeroOutMin=[]  ClampingZeroOutMax=[]  FilterDenConstantOutDataTypeStr=Inherit: Inherit via back propagation  FilterDenConstantOutMin=[]  FilterDenConstantOutMax=[]  PCopyOutDataTypeStr=Inherit: Inherit via back propagation  PCopyOutMin=[]  PCopyOutMax=[]  NCopyOutDataTypeStr=Inherit: Inherit via back propagation  NCopyOutMin=[]  NCopyOutMax=[]  IntegratorContinuousStateAttributes=''  IntegratorStateMustResolveToSignalObject=off  IntegratorRTWStateStorageClass=Auto  FilterContinuousStateAttributes=''  FilterStateMustResolveToSignalObject=off  FilterRTWStateStorageClass=Auto  ParallelPVariant=InternalParameters  IdealPVariant=Disabled  IVariant=InternalParameters  DVariant=InternalParameters  IntegratorVariant=Discrete  SatVariant=Enabled  AWVariant=Passthrough  PCopyVariant=Disabled  TRVariant=Disabled  FdbkBlocksVariant=Forward  IdealPFdbkVariant=Disabled  SatFdbkVariant=Disabled  DerivativeFilterVariant=ForwardEulerFilter  NVariant=InternalParameters  NCopyVariant=Disabled  FilterICVariant=InternalICsFilter  IntegratorICVariant=InternalICs  ExternalResetVariant=Disabled  TRSumVariant=Passthrough  SumFdbkVariant=Disabled  SumVariant=Sum_PID  TsampFilterVariant=InternalTs  TsampNgainVariant=Passthrough  TsampIntegralVariant=Passthrough  ExternalSaturationOutDataTypeStr=Inherit: Same as second input
  Product : Product  Inputs=3
  Rate Limiter : RateLimiter  RisingSlewLimit=MAX_DTHETA_DRIVER  FallingSlewLimit=-MAX_DTHETA_DRIVER  SampleTimeMode=inherited
  Saturation Dynamic : simulink/Discontinuities/Saturation Dynamic  OutMin=[]  OutMax=[]  OutDataTypeStr=Inherit: Same as second input  OutDataType=fixdt(1, 16)  OutScaling=2^-10  DoSatur=off
  Saturation2 : Saturate  UpperLimit=CENTER_STEER_ANGLE_MAX  LowerLimit=-CENTER_STEER_ANGLE_MAX
  Sign : Signum
  Sum : Sum  Inputs=|++
  Switch : Switch  Criteria=u2 ~= 0  SaturateOnIntegerOverflow=off  InputSameDT=off
  Switch1 : Switch  Criteria=u2 ~= 0  SaturateOnIntegerOverflow=off  InputSameDT=off
  To Workspace : ToWorkspace  VariableName=lookup_steering  SaveFormat=Timeseries  SampleTime=-1
  steering_angle : Outport
  wires:
  Saturation2/1 -> steering_angle/1
  Rate Limiter/1 -> Saturation2/1
  Switch/1 -> Switch1/1
  Controller Information/1 -> Bus Selector/1
  Bus Selector/3 -> Sign/1, Abs/1  "<yaw_ref>"
  Bus Selector/4 -> 2-D Lookup Table1/2, 2-D Lookup Table2/2  "<v_cog>"
  2-D Lookup Table1/1 -> Min/1
  2-D Lookup Table2/1 -> Min/2
  Min/1 -> Product/3
  Bus Selector/1 -> PID Controller1/1, PID Controller2/1, PID Controller/1  "<p_error>"
  Product/1 -> To Workspace/1, Sum/2
  Saturation Dynamic/1 -> 2-D Lookup Table1/1, 2-D Lookup Table2/1
  Bus Selector/2 -> GreaterThan/1, 1-D Lookup Table/1  "<Vnow>"
  Abs/1 -> Saturation Dynamic/3, Saturation Dynamic/2
  1-D Lookup Table/1 -> Saturation Dynamic/1
  PID Controller/1 -> Switch/3
  PID Controller1/1 -> Switch/1
  Constant/1 -> GreaterThan/2
  Sign/1 -> GreaterThan1/1, Switch/2, Product/2
  Switch1/1 -> Sum/1
  PID Controller2/1 -> Switch1/3
  Constant1/1 -> GreaterThan1/2
  GreaterThan/1 -> NOT/1, NAND/1
  GreaterThan1/1 -> NAND/2
  NAND/1 -> Switch1/2
  NOT/1 -> Product/1
  Sum/1 -> Rate Limiter/1
